simulink model "vloop_test2"  (Simulink 8.4)
settings: Solver=ode15s  StartTime=0.0  StopTime=1.0  RelTol=1e-3
InitFcn:
  | G = 107.815;
libraries: roblocks x1
settings Model: Creator=pic  LastModifiedBy=corkep
settings SFSimCC: SimCustomInitializer=|
  | if ~exist(tau_d)
  |    tau_d = 0
  | end

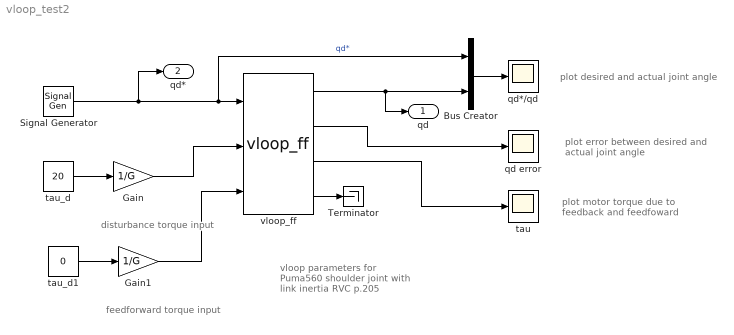
== system vloop_test2 ==
  note: plot motor torque due
      | to feedback and feedfoward
  note: plot error between desired and
      | actual joint angle
  note: plot desired and actual joint angle
  note: disturbance torque input
  note: feedforward torque input
  note: vloop parameters for
      | Puma560 shoulder joint
      | with link inertia
      | RVC p.205
  Bus Creator : BusCreator  Inputs=2
  Gain : Gain  Gain=1/G
  Gain1 : Gain  Gain=1/G
  Signal Generator : SignalGenerator  WaveForm=sawtooth  Frequency=2
  Terminator : Terminator
  qd error : Scope
      settings: TimeRange=1  YMin=0  YMax=0.7  SaveName=ScopeData2
  qd*/qd : Scope
      settings: TimeRange=1  YMin=0  YMax=90
  tau : Scope
      settings: TimeRange=1  YMin=-0.1  YMax=0.175
  tau_d : Constant  Value=20
  tau_d1 : Constant  Value=0
  vloop_ff : roblocks/Dynamics/vloop_ff  J=372e-6  B=817e-6  Km=0.228  tau_max=0.9  Kv=1  Ki=0  T=0.001
  qd : Outport
  qd* : Outport  Port=2
  wires:
  Signal Generator/1 -> qd*/1, vloop_ff/1, Bus Creator/1  "qd*"
  Bus Creator/1 -> qd*/qd/1
  tau_d/1 -> Gain/1
  vloop_ff/1 -> qd/1, Bus Creator/2
  vloop_ff/2 -> qd error/1
  Gain/1 -> vloop_ff/2
  vloop_ff/3 -> tau/1
  vloop_ff/4 -> Terminator/1
  tau_d1/1 -> Gain1/1
  Gain1/1 -> vloop_ff/3
